simulink model "Model4"  (R2019b)
settings: Solver=VariableStepAuto  StartTime=0.0  StopTime=time  RelTol=1e-3
values from neighbouring files (symbols this model uses):
  breath = 60/f    (= 3)    [Model_main.m]
  E1 = 16    [Model_main.m]
  E2 = 8    [Model_main.m]
  E_high = 100000    [Model_main.m]
  E_th = 5    [Model_main.m]
  insptime = (ieratio(1)/(ieratio(1)+ieratio(2)))*100    [Model_main.m]
  Pcontrol = 15    [Model_main.m]
  PEEP = 5    [Model_main.m]
  R = 10    [Model_main.m]
  R1 = 15    [Model_main.m]
  R2 = 10    [Model_main.m]
  TOP1 = 0    [Model_main.m]
  TOP2 = 5    [Model_main.m]
  V0 = 2    [Model_main.m]
  V0_th = 4.6    [Model_main.m]
libraries: simulink x1
settings Model: Creator=Amne  LastModifiedBy=Amne
settings SolverCC: ZeroCrossAlgorithm=Adaptive  AlgebraicLoopSolver=LineSearch
settings DataIOCC: ReturnWorkspaceOutputs=off
settings DebuggingCC: RTPrefix=warning  SignalRangeChecking=warning  IgnoredZcDiagnostic=none  UnderSpecifiedDimensionMsg=error  ArithmeticOperatorsInVariantConditions=warning
settings SFSimCC: SimUseLocalCustomCode=off  CustomCodeUndefinedFunction=UseInterfaceOnly
settings RTWCC: RTWUseLocalCustomCode=off

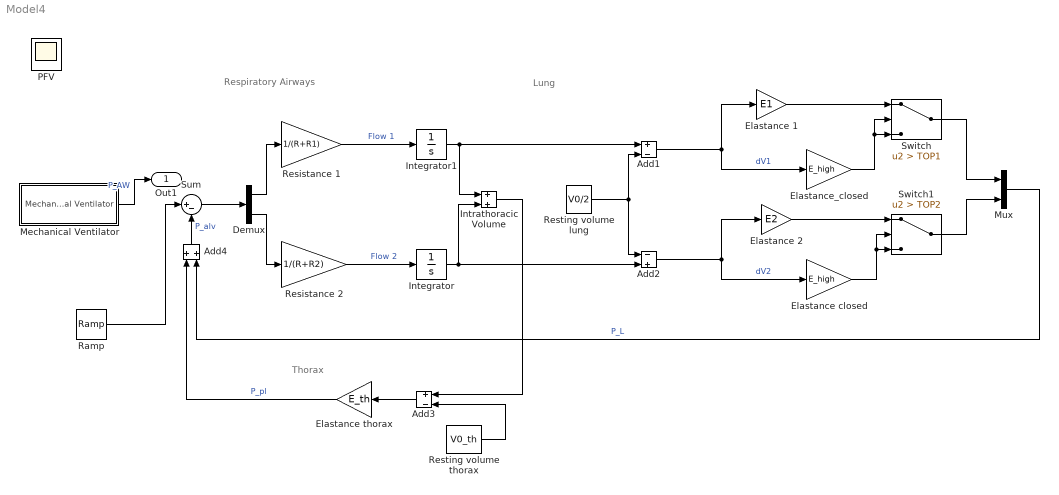
== system Model4 ==
  note: Lung
  note: Respiratory Airways
  note: Thorax
  Add1 : Sum  Inputs=+-
  Add2 : Sum  Inputs=-+
  Add3 : Sum  Inputs=+-
  Add4 : Sum
  Demux : Demux  Outputs=2
  Elastance 1 : Gain  Gain=E1
  "Elastance 2 " : Gain  Gain=E2
  Elastance closed : Gain  Gain=E_high
  Elastance thorax : Gain  Gain=E_th
  Elastance_closed : Gain  Gain=E_high
  Integrator : Integrator
  Integrator1 : Integrator
  Intrathoracic Volume : Sum
  "Mechanical Ventilator " : Subsystem
  Mux : Mux  Inputs=2
  Ramp : simulink/Sources/Ramp  slope=2  start=0  InitialOutput=-5
  Resistance 1 : Gain  Gain=1/(R+R1)
  Resistance 2 : Gain  Gain=1/(R+R2)
  "Resting volume lung " : Constant  Value=V0/2
  Resting volume thorax : Constant  Value=V0_th
  Sum : Sum  Inputs=|+-
  Switch : Switch  Criteria=u2 > Threshold  Threshold=TOP1
  Switch1 : Switch  Criteria=u2 > Threshold  Threshold=TOP2
  Out1 : Outport
  PFV : Scope
  wires:
  "Mechanical Ventilator "/1(Mechanical Ventilator) -> Out1/1  "P_AW"
  Resistance 1/1 -> Integrator1/1  "Flow 1"
  Elastance 1/1 -> Switch/1
  Mux/1 -> Add4/2  "P_L"
  Add2/1 -> Elastance closed/1, "Elastance 2 "/1  "dV2"
  Add1/1 -> Elastance_closed/1, Elastance 1/1  "dV1"
  Resting volume thorax/1 -> Add3/2
  Add3/1 -> Elastance thorax/1
  Elastance thorax/1 -> Add4/1  "P_pl"
  Add4/1 -> Sum/2  "P_alv"
  "Resting volume lung "/1 -> Add2/1, Add1/2
  Elastance_closed/1 -> Switch/3, Switch/2
  Switch/1 -> Mux/1
  "Elastance 2 "/1 -> Switch1/1
  Switch1/1 -> Mux/2
  Elastance closed/1 -> Switch1/2, Switch1/3
  Integrator/1 -> Add2/2, Intrathoracic Volume/2
  Sum/1 -> Demux/1
  Demux/1 -> Resistance 1/1
  Demux/2 -> Resistance 2/1
  Resistance 2/1 -> Integrator/1  "Flow 2"
  Integrator1/1 -> Add1/1, Intrathoracic Volume/1
  Intrathoracic Volume/1 -> Add3/1
  Ramp/1 -> Sum/1

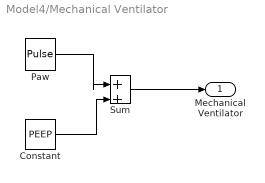
== system Model4/Mechanical Ventilator  ==
  Constant : Constant  Value=PEEP  SampleTime=0.1
  Paw : DiscretePulseGenerator  PulseType=Time based  Amplitude=Pcontrol  Period=breath  PulseWidth=insptime  PhaseDelay=2  SampleTime=0.1
  Sum : Sum  Inputs=|++
  Mechanical Ventilator : Outport  VectorParamsAs1DForOutWhenUnconnected=off
  wires:
  Paw/1 -> Sum/1
  Constant/1 -> Sum/2
  Sum/1 -> Mechanical Ventilator/1
